simulink model "Exp2"  (R2018a)
settings: Solver=FixedStepAuto  StartTime=0.0  StopTime=Inf  FixedStep=0.1  RelTol=1e-3  EnableMultiTasking=on
libraries: simulink x2, arduinolib x2
settings Model: SimulationMode=external  ExtModeTrigDuration=2  Creator=isuf  LastModifiedBy=user
settings OptimizationCC: MaxStackSize=64
settings DebuggingCC: ParameterTunabilityLossMsg=error
settings HardwareCC: ProdBitPerInt=16  ProdBitPerPointer=16  ProdBitPerSizeT=16  ProdBitPerPtrDiffT=16  ProdLargestAtomicFloat=None  ProdWordSize=8  ProdHWDeviceType=Atmel->AVR  UseEmbeddedCoderFeatures=off  UseSimulinkCoderFeatures=off
settings RTWCC: SystemTargetFile=ert.tlc  HardwareBoard=Arduino Mega 2560  TLCOptions=-aInlineSetEventsForThisBaseRateFcn=TLC_FALSE -aSuppressMultiTaskScheduler=TLC_FALSE -aRateBasedStepFcn=1  TemplateMakefile=ert_default_tmf  GenerateReport=on  Toolchain=Arduino AVR  BuildConfiguration=Faster Runs  LaunchReport=on
settings CodeAppCC: ForceParamTrailComments=on  OperatorAnnotations=on  StateflowObjectComments=on  MATLABSourceComments=on
settings ERTTargetCC: MultiwordLength=2048  ERTCustomFileBanners=off  SupportContinuousTime=on  SupportNonInlinedSFcns=on  RemoveResetFunc=off  SupportVariableSizeSignals=on  ModelStepFunctionPrototypeControlCompliant=off

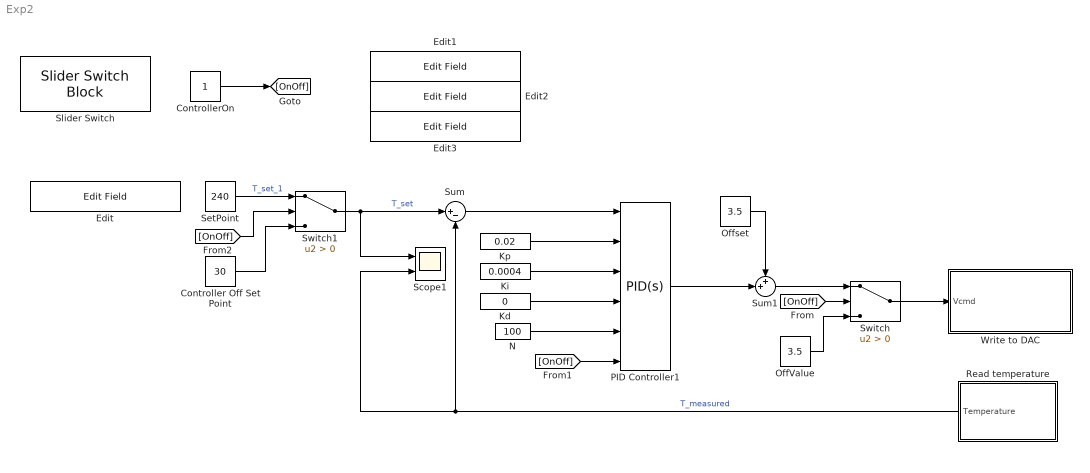
== system Exp2 ==
  Controller Off Set Point : Constant  Value=30
  ControllerOn : Constant
  Edit : EditField  WebBlockId=93  LabelPosition=Bottom  Alignment=Center
  Edit1 : EditField  WebBlockId=103  LabelPosition=Bottom  Alignment=Center
  Edit2 : EditField  WebBlockId=104  LabelPosition=Bottom  Alignment=Center
  Edit3 : EditField  WebBlockId=105  LabelPosition=Bottom  Alignment=Center
  Kd : Constant  Value=0
  Ki : Constant  Value=0.0004
  Kp : Constant  Value=0.02
  N : Constant  Value=100
  OffValue : Constant  Value=3.5
  Offset : Constant  Value=3.5
  PID Controller1 : simulink/Continuous/PID Controller  Controller=PID  TimeDomain=Continuous-time  SampleTime=-1  IntegratorMethod=Forward Euler  FilterMethod=Forward Euler  Form=Parallel  UseFilter=on  ControllerParametersSource=external  P=0.02  I=0.0005  D=0  N=100  InitialConditionSource=internal  InitialConditionForIntegrator=0  InitialConditionForFilter=0  ExternalReset=rising  LimitOutput=on  UpperSaturationLimit=1.5  LowerSaturationLimit=-1.5  LinearizeAsGain=on  AntiWindupMode=none  Kb=1  TrackingMode=off  Kt=1  PParamMin=[]  PParamMax=[]  IParamMin=[]  IParamMax=[]  DParamMin=[]  DParamMax=[]  NParamMin=[]  NParamMax=[]  KbParamMin=[]  KbParamMax=[]  KtParamMin=[]  KtParamMax=[]  POutMin=[]  POutMax=[]  IOutMin=[]  IOutMax=[]  DOutMin=[]  DOutMax=[]  NOutMin=[]  NOutMax=[]  KbOutMin=[]  KbOutMax=[]  KtOutMin=[]  KtOutMax=[]  IntegratorOutMin=[]  IntegratorOutMax=[]  FilterOutMin=[]  FilterOutMax=[]  SumOutMin=[]  SumOutMax=[]  SumI1OutMin=[]  SumI1OutMax=[]  SumI2OutMin=[]  SumI2OutMax=[]  SumI3OutMin=[]  SumI3OutMax=[]  SumDOutMin=[]  SumDOutMax=[]  SaturationOutMin=[]  SaturationOutMax=[]  IntegratorContinuousStateAttributes=''  IntegratorStateMustResolveToSignalObject=off  IntegratorRTWStateStorageClass=Auto  FilterContinuousStateAttributes=''  FilterStateMustResolveToSignalObject=off  FilterRTWStateStorageClass=Auto  DifferentiatorICPrevScaledInput=0  DifferentiatorOutMin=[]  DifferentiatorOutMax=[]  InitialConditionSetting=State (most efficient)  FilterDiffOutCoefMin=[]  FilterDiffOutCoefMax=[]  SumDenOutMin=[]  SumDenOutMax=[]  SumNumOutMin=[]  SumNumOutMax=[]  ReciprocalOutMin=[]  ReciprocalOutMax=[]  DivideOutMin=[]  DivideOutMax=[]  TunerSelectOption=Transfer Function Based (PID Tuner App)
  Read temperature : Subsystem
  Scope1 : Scope  NumInputPorts=2
  SetPoint : Constant  Value=240
  Slider Switch : SliderSwitchBlock  WebBlockId=115
      settings: Values={{'Off', 'On'}, [0 1]}
  Sum : Sum  Inputs=|+-
  Sum1 : Sum  Inputs=++|
  Switch : Switch  Criteria=u2 > Threshold
  Switch1 : Switch  Criteria=u2 > Threshold
  Write to DAC : Subsystem
  wires:
  Read temperature/1(Temperature) -> Sum/2, Scope1/2  "T_measured"
  Sum/1 -> PID Controller1/1
  [OnOff] -> Switch/2
  OffValue/1 -> Switch/3
  PID Controller1/1 -> Sum1/2
  Offset/1 -> Sum1/1
  Sum1/1 -> Switch/1
  Switch/1 -> Write to DAC/1(Vcmd)
  Kp/1 -> PID Controller1/2
  Ki/1 -> PID Controller1/3
  Kd/1 -> PID Controller1/4
  N/1 -> PID Controller1/5
  ControllerOn/1 -> [OnOff]
  [OnOff] -> PID Controller1/6
  SetPoint/1 -> Switch1/1  "T_set_1"
  Switch1/1 -> Scope1/1, Sum/1  "T_set"
  Controller Off Set Point/1 -> Switch1/3
  [OnOff] -> Switch1/2

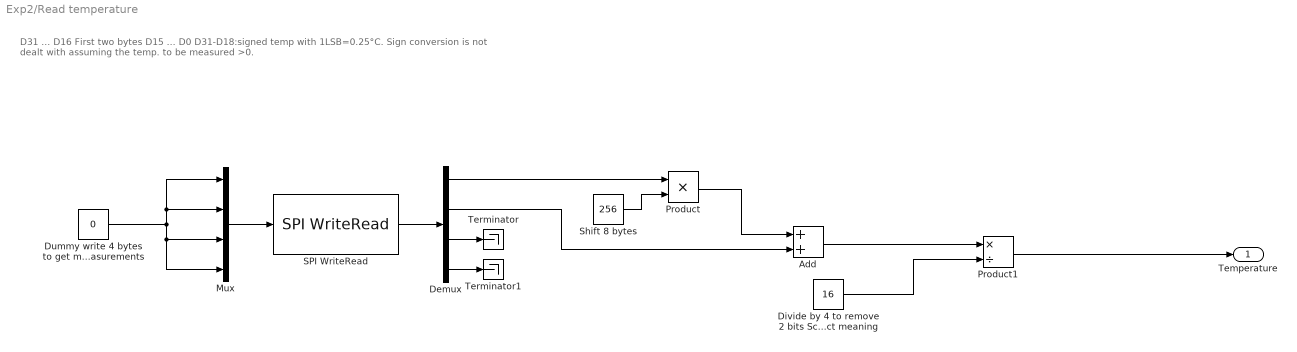
== system Exp2/Read temperature ==
  note: D31 ... D16 First two bytes
      | D15 ... D0
      |
      | D31-D18:signed temp with 1LSB=0.25°C. Sign conversion is not dealt with assuming the temp. to be measured >0.
  Add : Sum  OutDataTypeStr=uint32
  Demux : Demux
  Divide by 4 to remove 2 bits Scale by 0.25 (Divide by 4) to obtain the correct meaning : Constant  Value=16  OutDataTypeStr=uint8
  Dummy write 4 bytes to get measurements : Constant  Value=0  OutDataTypeStr=uint8
  Mux : Mux
  Product : Product  OutDataTypeStr=uint32
  Product1 : Product  Inputs=*/  OutDataTypeStr=double
  SPI WriteRead : arduinolib/SPI WriteRead  slaveSelectPin_=53  blockPlatform=arduino
      settings: SourceProductName=Simulink Support Package for Arduino Hardware  SourceProductBaseCode=ARDUINO
  Shift 8 bytes : Constant  Value=256  OutDataTypeStr=uint16
  Terminator : Terminator
  Terminator1 : Terminator
  Temperature : Outport
  wires:
  Add/1 -> Product1/1
  Shift 8 bytes/1 -> Product/2
  Product/1 -> Add/1
  Divide by 4 to remove 2 bits Scale by 0.25 (Divide by 4) to obtain the correct meaning/1 -> Product1/2
  Product1/1 -> Temperature/1
  Demux/3 -> Terminator/1
  Mux/1 -> SPI WriteRead/1
  Dummy write 4 bytes to get measurements/1 -> Mux/1, Mux/2, Mux/4, Mux/3
  Demux/2 -> Add/2
  SPI WriteRead/1 -> Demux/1
  Demux/1 -> Product/1
  Demux/4 -> Terminator1/1

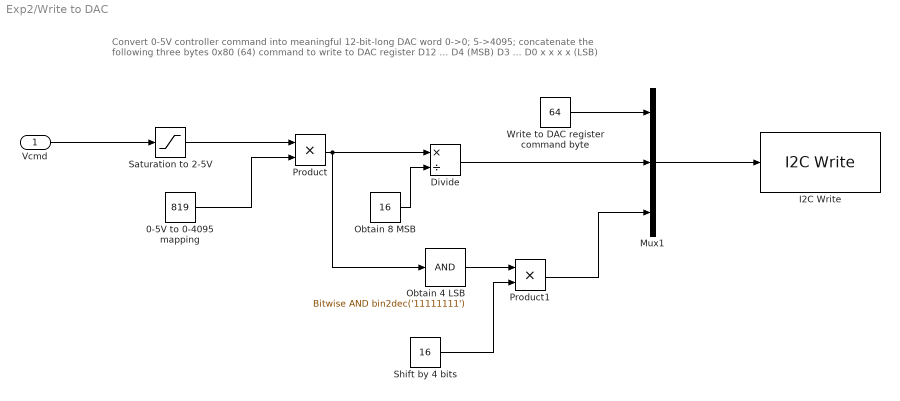
== system Exp2/Write to DAC ==
  note: Convert 0-5V controller command into meaningful 12-bit-long DAC word
      | 0->0; 5->4095; concatenate the following three bytes
      | 0x80 (64) command to write to DAC register
      | D12 ... D4 (MSB)
      | D3 ... D0 x x x x (LSB)
  Vcmd : Inport
  0-5V to 0-4095 mapping : Constant  Value=819  OutDataTypeStr=uint16
  Divide : Product  Inputs=*/  OutDataTypeStr=uint8
  I2C Write : arduinolib/I2C Write  SlaveAddress_=hex2dec( '60' )  RegisterAddressEnable=off  RegisterAddress_=hex2dec( '20' )  Datatype=uint8  ByteOrder=Big Endian  blockPlatform=arduino
      settings: SourceProductName=Simulink Support Package for Arduino Hardware  SourceProductBaseCode=ARDUINO
  Mux1 : Mux  Inputs=3
  Obtain 4 LSB : simulink/Logic and Bit Operations/Bitwise Operator  logicop=AND  UseBitMask=on  BitMask=bin2dec('11111111')  BitMaskRealWorld=Stored Integer
  "Obtain 8 MSB " : Constant  Value=16  OutDataTypeStr=uint8
  Product : Product  OutDataTypeStr=uint16
  Product1 : Product  OutDataTypeStr=uint8
  Saturation to 2-5V : Saturate  UpperLimit=5  LowerLimit=2
  Shift by 4 bits : Constant  Value=16  OutDataTypeStr=uint8
  Write to DAC register command byte : Constant  Value=64  OutDataTypeStr=uint8
  wires:
  Write to DAC register command byte/1 -> Mux1/1
  Saturation to 2-5V/1 -> Product/1
  0-5V to 0-4095 mapping/1 -> Product/2
  Vcmd/1 -> Saturation to 2-5V/1
  Mux1/1 -> I2C Write/1
  Obtain 4 LSB/1 -> Product1/1
  Product/1 -> Divide/1, Obtain 4 LSB/1
  Product1/1 -> Mux1/3
  "Obtain 8 MSB "/1 -> Divide/2
  Divide/1 -> Mux1/2
  Shift by 4 bits/1 -> Product1/2
